simulink model "centralized_FD_basic_01_2017b"  (R2017b)
settings: Solver=VariableStepAuto  StartTime=0.0  StopTime=Tstop  RelTol=1e-3
values from neighbouring files (symbols this model uses):
  faultMag = [0 0 1]    [ProblemData.m]
  faultTime = [1e6 1e6 400]    [ProblemData.m]
  Lambda = diag([0.91 0.91 0.91])    [ProblemData.m]
  noiseRange = [-peakNoise ; +peakNoise]    [ProblemData.m]
  pipeCoeff = [1 1 1]    [ProblemData.m]
  pipeCoeffN = makeParUncertain(pipeCoeff,uncRelative)    [ProblemData.m]
  pipeCross = [5 5 5]*1e-4    [ProblemData.m]
  pipeCrossN = makeParUncertain(pipeCross,uncRelative)    [ProblemData.m]
  pumpACMagRelative = [0.1 0.25]    [ProblemData.m]
  pumpACPeriod = [10 50]    [ProblemData.m]
  pumpDCMag = [1.5 1.5]*1e-3    [ProblemData.m]
  tankCross = [0.156 0.156 0.156]    [ProblemData.m]
  tankCrossN = makeParUncertain(tankCross,uncRelative)    [ProblemData.m]
  tankInit = [0 2.5 5]    [ProblemData.m]
  tankInitN = makeParUncertain(tankInit,uncRelative)    [ProblemData.m]
  tankMax = [10 10 10]    [ProblemData.m]
  tankMaxN = makeParUncertain(tankMax,uncRelative)    [ProblemData.m]
  tankMin = [0 0 0]    [ProblemData.m]
  tankMinN = tankMin    [ProblemData.m]
  Tdelay = 500    [ProblemData.m]
  Ts = 0.01    [ProblemData.m]
(part 1 of 2)
settings Model: Creator=riccardoferrar  LastModifiedBy=TUDelft SID

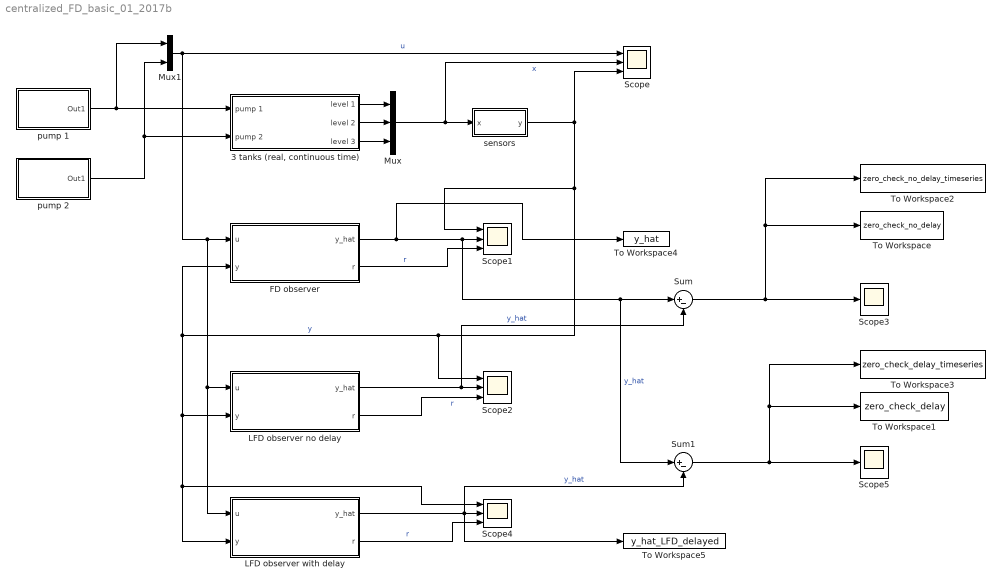
== system centralized_FD_basic_01_2017b ==
  "3 tanks (real, continuous time)" : Subsystem
  FD observer : Subsystem  SystemSampleTime=Ts
  LFD observer no delay : Subsystem  SystemSampleTime=Ts
  LFD observer with delay : Subsystem  SystemSampleTime=Ts
  Mux : Mux  Inputs=3
  Mux1 : Mux  Inputs=2
  Scope{,1..2,4} (4 alike) : Scope  NumInputPorts=3
  Scope3 : Scope
  Scope5 : Scope
  Sum : Sum  Inputs=|+-
  Sum1 : Sum  Inputs=|+-
  To Workspace : ToWorkspace  VariableName=zero_check_no_delay  SampleTime=-1
  To Workspace1 : ToWorkspace  VariableName=zero_check_delay  SampleTime=-1
  To Workspace2 : ToWorkspace  VariableName=zero_check_no_delay_timeseries  SaveFormat=Timeseries  SampleTime=-1
  To Workspace3 : ToWorkspace  VariableName=zero_check_delay_timeseries  SaveFormat=Timeseries  SampleTime=-1
  To Workspace4 : ToWorkspace  VariableName=y_hat  SaveFormat=Timeseries  SampleTime=-1
  To Workspace5 : ToWorkspace  VariableName=y_hat_LFD_delayed  SaveFormat=Timeseries  SampleTime=-1
  pump 1 : Subsystem  mask{pumpIdx=1}
      mask prompts: pumpIdx "Pump number"
  pump 2 : Subsystem  mask{pumpIdx=2}
      mask prompts: pumpIdx "Pump number"
  sensors : Subsystem
  wires:
  pump 1/1(Out1) -> "3 tanks (real, continuous time)"/1(pump 1), Mux1/1
  pump 2/1(Out1) -> Mux1/2, "3 tanks (real, continuous time)"/2(pump 2)
  "3 tanks (real, continuous time)"/1(level 1) -> Mux/1
  "3 tanks (real, continuous time)"/2(level 2) -> Mux/2
  "3 tanks (real, continuous time)"/3(level 3) -> Mux/3
  Mux1/1 -> LFD observer with delay/1(u), LFD observer no delay/1(u), FD observer/1(u), Scope/1  "u"
  sensors/1(y) -> Scope/3, Scope1/1, Scope2/1, Scope4/1, LFD observer with delay/2(y), LFD observer no delay/2(y), FD observer/2(y)  "y"
  FD observer/1(y_hat) -> To Workspace4/1, Sum1/1, Sum/1, Scope1/2  "y_hat"
  FD observer/2(r) -> Scope1/3  "r"
  Mux/1 -> Scope/2, sensors/1(x)  "x"
  LFD observer no delay/1(y_hat) -> Sum/2, Scope2/2  "y_hat"
  LFD observer no delay/2(r) -> Scope2/3  "r"
  Sum/1 -> To Workspace2/1, To Workspace/1, Scope3/1
  LFD observer with delay/1(y_hat) -> To Workspace5/1, Scope4/2, Sum1/2  "y_hat"
  LFD observer with delay/2(r) -> Scope4/3  "r"
  Sum1/1 -> To Workspace3/1, To Workspace1/1, Scope5/1

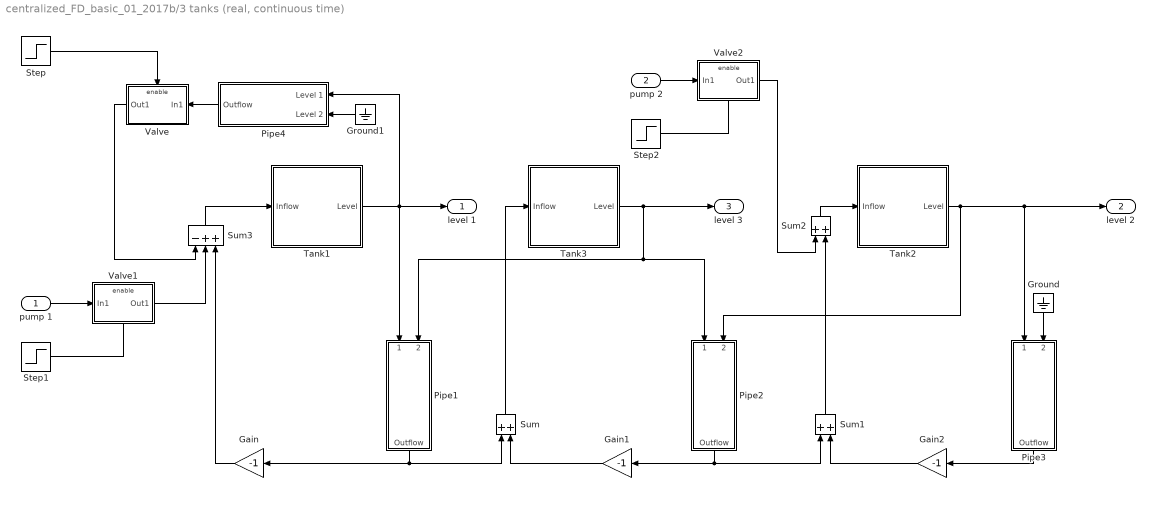
== system centralized_FD_basic_01_2017b/3 tanks (real, continuous time) ==
  pump 1 : Inport
  pump 2 : Inport  Port=2
  Gain : Gain  Gain=-1
  Gain1 : Gain  Gain=-1
  Gain2 : Gain  Gain=-1
  Ground : Ground
  Ground1 : Ground
  Pipe1 : Subsystem  mask(Connection Pipe){S_p=pipeCross(1), c_o=pipeCoeff(1)}
      mask prompts: S_p "Pipe cross-section [m^2]"; c_o "Outflow coefficient"
      mask help:
      | Connection pipe between two tanks.
      | The pipe cross-section and the outflow coefficient are mask block parameters.
      mask Help:
      | Enter the pipe cross-section [S_p] and the outflow coefficient [c_o] in the block dialog parameter fields.
      | 
      | The block generates the pipe's flow-rate. The input signals are the level of fluid into both the tanks, connected by the pipe. If the level in the first tank is bigger than the level in the second one, the fluid flow from the first to the second tank, else in the opposite way.
      mask Display: image(imread('pipe.jpg'));
  Pipe2 : Subsystem  mask(Connection Pipe){S_p=pipeCross(2), c_o=pipeCoeff(2)}
      mask prompts: S_p "Pipe cross-section [m^2]"; c_o "Outflow coefficient"
      mask help:
      | Connection pipe between two tanks.
      | The pipe cross-section and the outflow coefficient are mask block parameters.
      mask Help:
      | Enter the pipe cross-section [S_p] and the outflow coefficient [c_o] in the block dialog parameter fields.
      | 
      | The block generates the pipe's flow-rate. The input signals are the level of fluid into both the tanks, connected by the pipe. If the level in the first tank is bigger than the level in the second one, the fluid flow from the first to the second tank, else in the opposite way.
      mask Display: image(imread('pipe.jpg'));
  Pipe3 : Subsystem  mask(Connection Pipe){S_p=pipeCross(3), c_o=pipeCoeff(3)}
      mask prompts: S_p "Pipe cross-section [m^2]"; c_o "Outflow coefficient"
      mask help:
      | Connection pipe between two tanks.
      | The pipe cross-section and the outflow coefficient are mask block parameters.
      mask Help:
      | Enter the pipe cross-section [S_p] and the outflow coefficient [c_o] in the block dialog parameter fields.
      | 
      | The block generates the pipe's flow-rate. The input signals are the level of fluid into both the tanks, connected by the pipe. If the level in the first tank is bigger than the level in the second one, the fluid flow from the first to the second tank, else in the opposite way.
      mask Display: image(imread('pipe.jpg'));
  Pipe4 : Subsystem  mask(Connection Pipe){S_p=faultMag(2), c_o=1}
      mask prompts: S_p "Pipe cross-section [m^2]"; c_o "Outflow coefficient"
      mask help:
      | Connection pipe between two tanks.
      | The pipe cross-section and the outflow coefficient are mask block parameters.
      mask Help:
      | Enter the pipe cross-section [S_p] and the outflow coefficient [c_o] in the block dialog parameter fields.
      | 
      | The block generates the pipe's flow-rate. The input signals are the level of fluid into both the tanks, connected by the pipe. If the level in the first tank is bigger than the level in the second one, the fluid flow from the first to the second tank, else in the opposite way.
      mask Display: image(imread('pipe.jpg'));
  Step : Step  Time=faultTime(2)  SampleTime=0
  Step1 : Step  Time=faultTime(1)  Before=1  After=1-faultMag(1)  SampleTime=0
  Step2 : Step  Time=faultTime(3)  Before=1  After=1-faultMag(3)  SampleTime=0
  Sum : Sum
  Sum1 : Sum
  Sum2 : Sum
  Sum3 : Sum  Inputs=-++
  Tank1 : Subsystem  mask(Tank system){S=tankCross(1), x_0=tankInit(1), max_level=tankMax(1), min_level=tankMin(1)}
      mask prompts: S "Tank cross-section [m^2]"; x_0 "Initial fluid level [m"; max_level "Maximum fluid level [m]"; min_level "Minimum fluid level [m]"
      mask help:
      | Model of  a simple tank system. The input is a fluid flow-rate (may be positive or negative), the output is the fluid level in the tank.
      |
      | The tank cross-section, the initial, minimum and maximum fluid level are mask block parameters.
      mask Help:
      | Enter the tank cross-section, the initial, minimum, maximum fluid level in the block dialog parameter fields.
      | 
      | The block models a simple tank system. The input is the fluid flow-rate (positive or negative) that feeds the system; the output is the fluid level in the tank.
      mask Display: image(imread('tank.jpg'));
  Tank2 : Subsystem  mask(Tank system){S=tankCross(2), x_0=tankInit(2), max_level=tankMax(2), min_level=tankMin(2)}
      mask prompts: S "Tank cross-section [m^2]"; x_0 "Initial fluid level [m"; max_level "Maximum fluid level [m]"; min_level "Minimum fluid level [m]"
      mask help:
      | Model of  a simple tank system. The input is a fluid flow-rate (may be positive or negative), the output is the fluid level in the tank.
      |
      | The tank cross-section, the initial, minimum and maximum fluid level are mask block parameters.
      mask Help:
      | Enter the tank cross-section, the initial, minimum, maximum fluid level in the block dialog parameter fields.
      | 
      | The block models a simple tank system. The input is the fluid flow-rate (positive or negative) that feeds the system; the output is the fluid level in the tank.
      mask Display: image(imread('tank.jpg'));
  Tank3 : Subsystem  mask(Tank system){S=tankCross(3), x_0=tankInit(3), max_level=tankMax(3), min_level=tankMin(3)}
      mask prompts: S "Tank cross-section [m^2]"; x_0 "Initial fluid level [m"; max_level "Maximum fluid level [m]"; min_level "Minimum fluid level [m]"
      mask help:
      | Model of  a simple tank system. The input is a fluid flow-rate (may be positive or negative), the output is the fluid level in the tank.
      |
      | The tank cross-section, the initial, minimum and maximum fluid level are mask block parameters.
      mask Help:
      | Enter the tank cross-section, the initial, minimum, maximum fluid level in the block dialog parameter fields.
      | 
      | The block models a simple tank system. The input is the fluid flow-rate (positive or negative) that feeds the system; the output is the fluid level in the tank.
      mask Display: image(imread('tank.jpg'));
  Valve : Subsystem  TreatAsAtomicUnit=on  mask(Valve subsystem){}
      mask help: Model of a valve. When the control signal is greather then 0, the output is equal to the input. Otherwise, the output is 0.
      mask Display: image(imread('valve.jpg'))
  Valve1 : Subsystem  TreatAsAtomicUnit=on  mask(Valve subsystem){}
      mask help: Model of a valve. When the control signal is greather then 0, the output is equal to the input. Otherwise, the output is 0.
      mask Display: image(imread('valve.jpg'))
  Valve2 : Subsystem  TreatAsAtomicUnit=on  mask(Valve subsystem){}
      mask help: Model of a valve. When the control signal is greather then 0, the output is equal to the input. Otherwise, the output is 0.
      mask Display: image(imread('valve.jpg'))
  level 1 : Outport
  level 2 : Outport  Port=2
  level 3 : Outport  Port=3
  wires:
  Sum/1 -> Tank3/1(Inflow)
  Gain1/1 -> Sum/2
  Pipe2/1(Outflow) -> Sum1/1, Gain1/1
  Gain/1 -> Sum3/3
  Tank2/1(Level) -> level 2/1, Pipe3/1(Level 1), Pipe2/2(Level 2)
  Sum1/1 -> Sum2/2
  Gain2/1 -> Sum1/2
  Pipe3/1(Outflow) -> Gain2/1
  Tank1/1(Level) -> Pipe1/1(Level 1), Pipe4/1(Level 1), level 1/1
  Tank3/1(Level) -> level 3/1, Pipe2/1(Level 1), Pipe1/2(Level 2)
  Pipe1/1(Outflow) -> Gain/1, Sum/1
  Valve2/1(Out1) -> Sum2/1
  Sum2/1 -> Tank2/1(Inflow)
  Sum3/1 -> Tank1/1(Inflow)
  Ground/1 -> Pipe3/2(Level 2)
  Ground1/1 -> Pipe4/2(Level 2)
  Pipe4/1(Outflow) -> Valve/1(In1)
  Valve/1(Out1) -> Sum3/1
  Step/1 -> Valve/Enable
  pump 1/1 -> Valve1/1(In1)
  Valve1/1(Out1) -> Sum3/2
  Step1/1 -> Valve1/Enable
  Step2/1 -> Valve2/Enable
  pump 2/1 -> Valve2/1(In1)

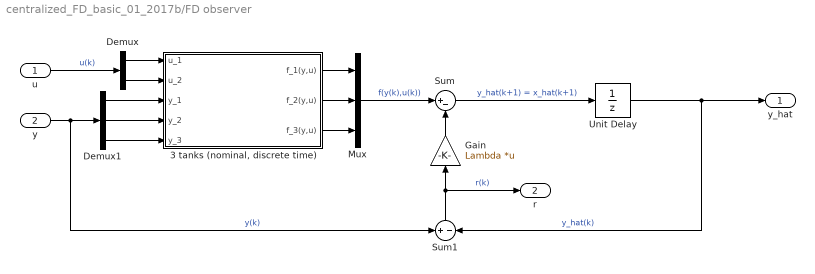
== system centralized_FD_basic_01_2017b/FD observer ==
  u : Inport
  y : Inport  Port=2
  "3 tanks (nominal, discrete time)" : Subsystem
  Demux : Demux  Outputs=2
  Demux1 : Demux  Outputs=3
  Gain : Gain  Gain=Lambda  Multiplication=Matrix(K*u)
  Mux : Mux  Inputs=3
  Sum : Sum  Inputs=|+-
  Sum1 : Sum  Inputs=+|-
  Unit Delay : UnitDelay  InitialCondition=tankInitN  SampleTime=-1
  y_hat : Outport
  r : Outport  Port=2
  wires:
  y/1 -> Sum1/1, Demux1/1  "y(k)"
  Demux1/3 -> "3 tanks (nominal, discrete time)"/5(y_3)
  u/1 -> Demux/1  "u(k)"
  Demux1/2 -> "3 tanks (nominal, discrete time)"/4(y_2)
  Demux/2 -> "3 tanks (nominal, discrete time)"/2(u_2)
  Demux1/1 -> "3 tanks (nominal, discrete time)"/3(y_1)
  Demux/1 -> "3 tanks (nominal, discrete time)"/1(u_1)
  "3 tanks (nominal, discrete time)"/1(f_1(y,u)) -> Mux/1
  "3 tanks (nominal, discrete time)"/2(f_2(y,u)) -> Mux/2
  "3 tanks (nominal, discrete time)"/3(f_3(y,u)) -> Mux/3
  Mux/1 -> Sum/1  "f(y(k),u(k))"
  Sum/1 -> Unit Delay/1  "y_hat(k+1) = x_hat(k+1)"
  Unit Delay/1 -> y_hat/1, Sum1/2  "y_hat(k)"
  Sum1/1 -> r/1, Gain/1  "r(k)"
  Gain/1 -> Sum/2

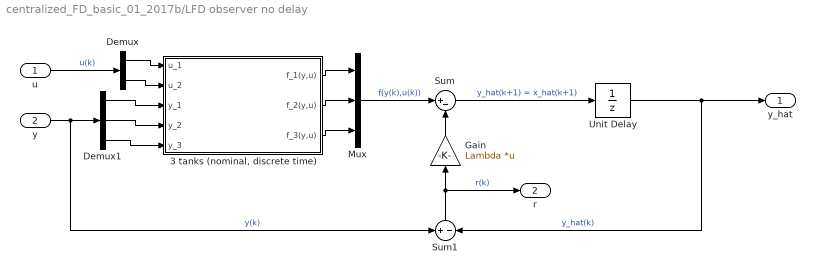
== system centralized_FD_basic_01_2017b/LFD observer no delay ==
  u : Inport
  y : Inport  Port=2
  "3 tanks (nominal, discrete time)" : Subsystem
  Demux : Demux  Outputs=2
  Demux1 : Demux  Outputs=3
  Gain : Gain  Gain=Lambda  Multiplication=Matrix(K*u)
  Mux : Mux  Inputs=3
  Sum : Sum  Inputs=|+-
  Sum1 : Sum  Inputs=+|-
  Unit Delay : UnitDelay  InitialCondition=tankInitN  SampleTime=-1
  y_hat : Outport
  r : Outport  Port=2
  wires:
  y/1 -> Sum1/1, Demux1/1  "y(k)"
  Demux1/3 -> "3 tanks (nominal, discrete time)"/5(y_3)
  u/1 -> Demux/1  "u(k)"
  Demux1/2 -> "3 tanks (nominal, discrete time)"/4(y_2)
  Demux/2 -> "3 tanks (nominal, discrete time)"/2(u_2)
  Demux1/1 -> "3 tanks (nominal, discrete time)"/3(y_1)
  Demux/1 -> "3 tanks (nominal, discrete time)"/1(u_1)
  "3 tanks (nominal, discrete time)"/1(f_1(y,u)) -> Mux/1
  "3 tanks (nominal, discrete time)"/2(f_2(y,u)) -> Mux/2
  "3 tanks (nominal, discrete time)"/3(f_3(y,u)) -> Mux/3
  Mux/1 -> Sum/1  "f(y(k),u(k))"
  Sum/1 -> Unit Delay/1  "y_hat(k+1) = x_hat(k+1)"
  Unit Delay/1 -> y_hat/1, Sum1/2  "y_hat(k)"
  Sum1/1 -> r/1, Gain/1  "r(k)"
  Gain/1 -> Sum/2

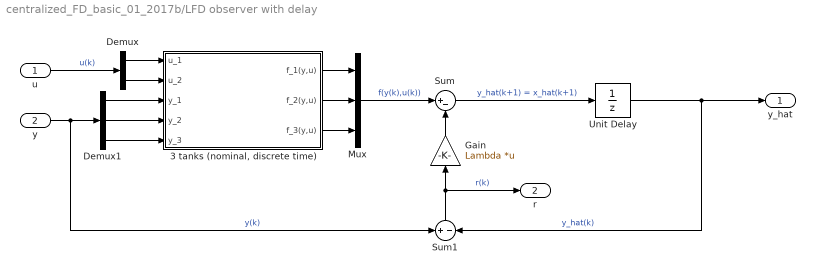
== system centralized_FD_basic_01_2017b/LFD observer with delay ==
  u : Inport
  y : Inport  Port=2
  "3 tanks (nominal, discrete time)" : Subsystem
  Demux : Demux  Outputs=2
  Demux1 : Demux  Outputs=3
  Gain : Gain  Gain=Lambda  Multiplication=Matrix(K*u)
  Mux : Mux  Inputs=3
  Sum : Sum  Inputs=|+-
  Sum1 : Sum  Inputs=+|-
  Unit Delay : UnitDelay  InitialCondition=tankInitN  SampleTime=-1
  y_hat : Outport
  r : Outport  Port=2
  wires:
  y/1 -> Sum1/1, Demux1/1  "y(k)"
  Demux1/3 -> "3 tanks (nominal, discrete time)"/5(y_3)
  u/1 -> Demux/1  "u(k)"
  Demux1/2 -> "3 tanks (nominal, discrete time)"/4(y_2)
  Demux/2 -> "3 tanks (nominal, discrete time)"/2(u_2)
  Demux1/1 -> "3 tanks (nominal, discrete time)"/3(y_1)
  Demux/1 -> "3 tanks (nominal, discrete time)"/1(u_1)
  "3 tanks (nominal, discrete time)"/1(f_1(y,u)) -> Mux/1
  "3 tanks (nominal, discrete time)"/2(f_2(y,u)) -> Mux/2
  "3 tanks (nominal, discrete time)"/3(f_3(y,u)) -> Mux/3
  Mux/1 -> Sum/1  "f(y(k),u(k))"
  Sum/1 -> Unit Delay/1  "y_hat(k+1) = x_hat(k+1)"
  Unit Delay/1 -> y_hat/1, Sum1/2  "y_hat(k)"
  Sum1/1 -> r/1, Gain/1  "r(k)"
  Gain/1 -> Sum/2

== system centralized_FD_basic_01_2017b/pump 1 ==
  Bias : Bias  Bias=1
  Product : Product
  Signal Generator : SignalGenerator  Amplitude=pumpACMagRelative(pumpIdx)  Frequency=1/pumpACPeriod(pumpIdx)  Units=rad/sec
  pump 1 : Constant  Value=pumpDCMag(pumpIdx)
  Out1 : Outport
  wires:
  Product/1 -> Out1/1
  Bias/1 -> Product/1
  pump 1/1 -> Product/2
  Signal Generator/1 -> Bias/1

== system centralized_FD_basic_01_2017b/pump 2 ==
  Bias : Bias  Bias=1
  Product : Product
  Signal Generator : SignalGenerator  Amplitude=pumpACMagRelative(pumpIdx)  Frequency=1/pumpACPeriod(pumpIdx)  Units=rad/sec
  pump 1 : Constant  Value=pumpDCMag(pumpIdx)
  Out1 : Outport
  wires:
  Product/1 -> Out1/1
  Bias/1 -> Product/1
  pump 1/1 -> Product/2
  Signal Generator/1 -> Bias/1

== system centralized_FD_basic_01_2017b/sensors ==
  x : Inport
  Sum : Sum  Inputs=|++
  Uniform Random Number : UniformRandomNumber  Minimum=noiseRange(1,:)  Maximum=noiseRange(2,:)  SampleTime=Ts
  y : Outport
  wires:
  Sum/1 -> y/1
  Uniform Random Number/1 -> Sum/2
  x/1 -> Sum/1

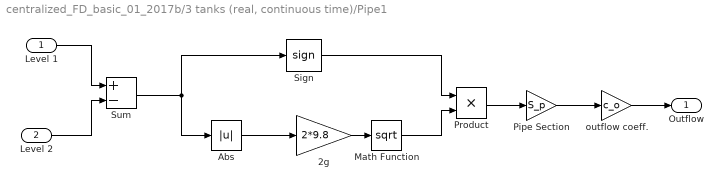
== system centralized_FD_basic_01_2017b/3 tanks (real, continuous time)/Pipe1 ==
  Level 1 : Inport
  Level 2 : Inport  Port=2
  2g : Gain  Gain=2*9.8  SaturateOnIntegerOverflow=on  OutDataTypeStr=Inherit: Same as input  ParamDataTypeStr=Inherit: Same as input
  Abs : Abs  SaturateOnIntegerOverflow=on
  Math Function : Math  Operator=sqrt  SaturateOnIntegerOverflow=on
  Pipe Section : Gain  Gain=S_p  SaturateOnIntegerOverflow=on  OutDataTypeStr=Inherit: Same as input  ParamDataTypeStr=Inherit: Same as input
  Product : Product  SaturateOnIntegerOverflow=on  InputSameDT=on  OutDataTypeStr=Inherit: Same as first input
  Sign : Signum
  Sum : Sum  Inputs=+-  SaturateOnIntegerOverflow=on  InputSameDT=on  OutDataTypeStr=Inherit: Same as first input
  outflow coeff. : Gain  Gain=c_o  SaturateOnIntegerOverflow=on  OutDataTypeStr=Inherit: Same as input  ParamDataTypeStr=Inherit: Same as input
  Outflow : Outport
  wires:
  outflow coeff./1 -> Outflow/1
  Pipe Section/1 -> outflow coeff./1
  Product/1 -> Pipe Section/1
  Sign/1 -> Product/1
  Math Function/1 -> Product/2
  2g/1 -> Math Function/1
  Abs/1 -> 2g/1
  Sum/1 -> Abs/1, Sign/1
  Level 2/1 -> Sum/2
  Level 1/1 -> Sum/1

== system centralized_FD_basic_01_2017b/3 tanks (real, continuous time)/Pipe2 ==
  Level 1 : Inport
  Level 2 : Inport  Port=2
  2g : Gain  Gain=2*9.8  SaturateOnIntegerOverflow=on  OutDataTypeStr=Inherit: Same as input  ParamDataTypeStr=Inherit: Same as input
  Abs : Abs  SaturateOnIntegerOverflow=on
  Math Function : Math  Operator=sqrt  SaturateOnIntegerOverflow=on
  Pipe Section : Gain  Gain=S_p  SaturateOnIntegerOverflow=on  OutDataTypeStr=Inherit: Same as input  ParamDataTypeStr=Inherit: Same as input
  Product : Product  SaturateOnIntegerOverflow=on  InputSameDT=on  OutDataTypeStr=Inherit: Same as first input
  Sign : Signum
  Sum : Sum  Inputs=+-  SaturateOnIntegerOverflow=on  InputSameDT=on  OutDataTypeStr=Inherit: Same as first input
  outflow coeff. : Gain  Gain=c_o  SaturateOnIntegerOverflow=on  OutDataTypeStr=Inherit: Same as input  ParamDataTypeStr=Inherit: Same as input
  Outflow : Outport
  wires:
  outflow coeff./1 -> Outflow/1
  Pipe Section/1 -> outflow coeff./1
  Product/1 -> Pipe Section/1
  Sign/1 -> Product/1
  Math Function/1 -> Product/2
  2g/1 -> Math Function/1
  Abs/1 -> 2g/1
  Sum/1 -> Abs/1, Sign/1
  Level 2/1 -> Sum/2
  Level 1/1 -> Sum/1

== system centralized_FD_basic_01_2017b/3 tanks (real, continuous time)/Pipe3 ==
  Level 1 : Inport
  Level 2 : Inport  Port=2
  2g : Gain  Gain=2*9.8  SaturateOnIntegerOverflow=on  OutDataTypeStr=Inherit: Same as input  ParamDataTypeStr=Inherit: Same as input
  Abs : Abs  SaturateOnIntegerOverflow=on
  Math Function : Math  Operator=sqrt  SaturateOnIntegerOverflow=on
  Pipe Section : Gain  Gain=S_p  SaturateOnIntegerOverflow=on  OutDataTypeStr=Inherit: Same as input  ParamDataTypeStr=Inherit: Same as input
  Product : Product  SaturateOnIntegerOverflow=on  InputSameDT=on  OutDataTypeStr=Inherit: Same as first input
  Sign : Signum
  Sum : Sum  Inputs=+-  SaturateOnIntegerOverflow=on  InputSameDT=on  OutDataTypeStr=Inherit: Same as first input
  outflow coeff. : Gain  Gain=c_o  SaturateOnIntegerOverflow=on  OutDataTypeStr=Inherit: Same as input  ParamDataTypeStr=Inherit: Same as input
  Outflow : Outport
  wires:
  outflow coeff./1 -> Outflow/1
  Pipe Section/1 -> outflow coeff./1
  Product/1 -> Pipe Section/1
  Sign/1 -> Product/1
  Math Function/1 -> Product/2
  2g/1 -> Math Function/1
  Abs/1 -> 2g/1
  Sum/1 -> Abs/1, Sign/1
  Level 2/1 -> Sum/2
  Level 1/1 -> Sum/1

== system centralized_FD_basic_01_2017b/3 tanks (real, continuous time)/Pipe4 ==
  Level 1 : Inport
  Level 2 : Inport  Port=2
  2g : Gain  Gain=2*9.8  SaturateOnIntegerOverflow=on  OutDataTypeStr=Inherit: Same as input  ParamDataTypeStr=Inherit: Same as input
  Abs : Abs  SaturateOnIntegerOverflow=on
  Math Function : Math  Operator=sqrt  SaturateOnIntegerOverflow=on
  Pipe Section : Gain  Gain=S_p  SaturateOnIntegerOverflow=on  OutDataTypeStr=Inherit: Same as input  ParamDataTypeStr=Inherit: Same as input
  Product : Product  SaturateOnIntegerOverflow=on  InputSameDT=on  OutDataTypeStr=Inherit: Same as first input
  Sign : Signum
  Sum : Sum  Inputs=+-  SaturateOnIntegerOverflow=on  InputSameDT=on  OutDataTypeStr=Inherit: Same as first input
  outflow coeff. : Gain  Gain=c_o  SaturateOnIntegerOverflow=on  OutDataTypeStr=Inherit: Same as input  ParamDataTypeStr=Inherit: Same as input
  Outflow : Outport
  wires:
  outflow coeff./1 -> Outflow/1
  Pipe Section/1 -> outflow coeff./1
  Product/1 -> Pipe Section/1
  Sign/1 -> Product/1
  Math Function/1 -> Product/2
  2g/1 -> Math Function/1
  Abs/1 -> 2g/1
  Sum/1 -> Abs/1, Sign/1
  Level 2/1 -> Sum/2
  Level 1/1 -> Sum/1

== system centralized_FD_basic_01_2017b/3 tanks (real, continuous time)/Tank1 ==
  Inflow : Inport
  Initial Level : Constant  Value=x_0
  Integrator : Integrator  InitialConditionSource=external  LimitOutput=on  UpperSaturationLimit=max_level  LowerSaturationLimit=min_level
  Tank Section : Gain  Gain=1/S  SaturateOnIntegerOverflow=on  OutDataTypeStr=Inherit: Same as input  ParamDataTypeStr=Inherit: Same as input
  Level : Outport  InitialOutput=0
  wires:
  Integrator/1 -> Level/1
  Initial Level/1 -> Integrator/2
  Tank Section/1 -> Integrator/1
  Inflow/1 -> Tank Section/1

== system centralized_FD_basic_01_2017b/3 tanks (real, continuous time)/Tank2 ==
  Inflow : Inport
  Initial Level : Constant  Value=x_0
  Integrator : Integrator  InitialConditionSource=external  LimitOutput=on  UpperSaturationLimit=max_level  LowerSaturationLimit=min_level
  Tank Section : Gain  Gain=1/S  SaturateOnIntegerOverflow=on  OutDataTypeStr=Inherit: Same as input  ParamDataTypeStr=Inherit: Same as input
  Level : Outport  InitialOutput=0
  wires:
  Integrator/1 -> Level/1
  Initial Level/1 -> Integrator/2
  Tank Section/1 -> Integrator/1
  Inflow/1 -> Tank Section/1

== system centralized_FD_basic_01_2017b/3 tanks (real, continuous time)/Tank3 ==
  Inflow : Inport
  Initial Level : Constant  Value=x_0
  Integrator : Integrator  InitialConditionSource=external  LimitOutput=on  UpperSaturationLimit=max_level  LowerSaturationLimit=min_level
  Tank Section : Gain  Gain=1/S  SaturateOnIntegerOverflow=on  OutDataTypeStr=Inherit: Same as input  ParamDataTypeStr=Inherit: Same as input
  Level : Outport  InitialOutput=0
  wires:
  Integrator/1 -> Level/1
  Initial Level/1 -> Integrator/2
  Tank Section/1 -> Integrator/1
  Inflow/1 -> Tank Section/1

== system centralized_FD_basic_01_2017b/3 tanks (real, continuous time)/Valve ==
  In1 : Inport
  Enable : EnablePort  StatesWhenEnabling=reset  ShowOutputPort=on
  Product : Product  SaturateOnIntegerOverflow=on  InputSameDT=on  OutDataTypeStr=Inherit: Same as first input
  Saturation : Saturate  UpperLimit=1.0  LowerLimit=0.0
  Out1 : Outport  OutputWhenDisabled=reset  InitialOutput=0
  wires:
  Enable/1 -> Saturation/1
  Saturation/1 -> Product/1
  In1/1 -> Product/2
  Product/1 -> Out1/1

== system centralized_FD_basic_01_2017b/3 tanks (real, continuous time)/Valve1 ==
  In1 : Inport
  Enable : EnablePort  StatesWhenEnabling=reset  ShowOutputPort=on
  Product : Product  SaturateOnIntegerOverflow=on  InputSameDT=on  OutDataTypeStr=Inherit: Same as first input
  Saturation : Saturate  UpperLimit=1.0  LowerLimit=0.0
  Out1 : Outport  OutputWhenDisabled=reset  InitialOutput=0
  wires:
  Enable/1 -> Saturation/1
  Saturation/1 -> Product/1
  In1/1 -> Product/2
  Product/1 -> Out1/1

== system centralized_FD_basic_01_2017b/3 tanks (real, continuous time)/Valve2 ==
  In1 : Inport
  Enable : EnablePort  StatesWhenEnabling=reset  ShowOutputPort=on
  Product : Product  SaturateOnIntegerOverflow=on  InputSameDT=on  OutDataTypeStr=Inherit: Same as first input
  Saturation : Saturate  UpperLimit=1.0  LowerLimit=0.0
  Out1 : Outport  OutputWhenDisabled=reset  InitialOutput=0
  wires:
  Enable/1 -> Saturation/1
  Saturation/1 -> Product/1
  In1/1 -> Product/2
  Product/1 -> Out1/1

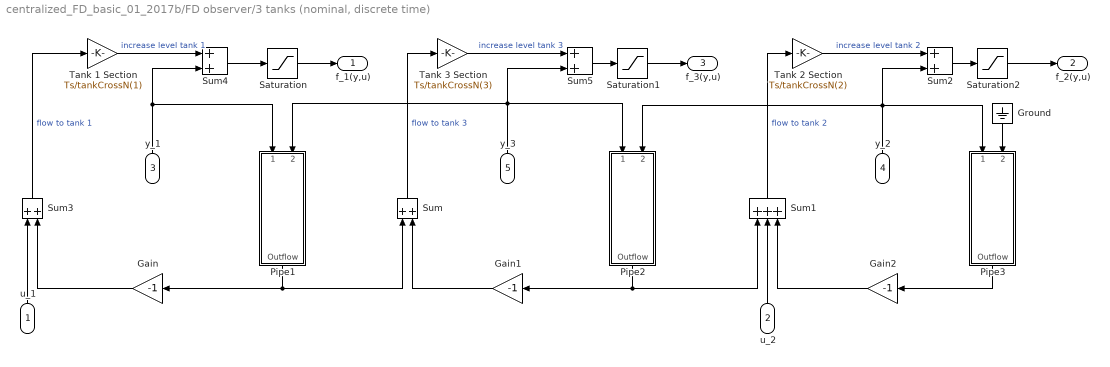
== system centralized_FD_basic_01_2017b/FD observer/3 tanks (nominal, discrete time) ==
  u_1 : Inport
  u_2 : Inport  Port=2
  y_1 : Inport  Port=3
  y_2 : Inport  Port=4
  y_3 : Inport  Port=5
  Gain : Gain  Gain=-1
  Gain1 : Gain  Gain=-1
  Gain2 : Gain  Gain=-1
  Ground : Ground
  Pipe1 : Subsystem  mask(Connection Pipe){S_p=pipeCrossN(1), c_o=pipeCoeffN(1)}
      mask prompts: S_p "Pipe cross-section [m^2]"; c_o "Outflow coefficient"
      mask help:
      | Connection pipe between two tanks.
      | The pipe cross-section and the outflow coefficient are mask block parameters.
      mask Help:
      | Enter the pipe cross-section [S_p] and the outflow coefficient [c_o] in the block dialog parameter fields.
      | 
      | The block generates the pipe's flow-rate. The input signals are the level of fluid into both the tanks, connected by the pipe. If the level in the first tank is bigger than the level in the second one, the fluid flow from the first to the second tank, else in the opposite way.
      mask Display: image(imread('pipe.jpg'));
  Pipe2 : Subsystem  mask(Connection Pipe){S_p=pipeCrossN(2), c_o=pipeCoeffN(2)}
      mask prompts: S_p "Pipe cross-section [m^2]"; c_o "Outflow coefficient"
      mask help:
      | Connection pipe between two tanks.
      | The pipe cross-section and the outflow coefficient are mask block parameters.
      mask Help:
      | Enter the pipe cross-section [S_p] and the outflow coefficient [c_o] in the block dialog parameter fields.
      | 
      | The block generates the pipe's flow-rate. The input signals are the level of fluid into both the tanks, connected by the pipe. If the level in the first tank is bigger than the level in the second one, the fluid flow from the first to the second tank, else in the opposite way.
      mask Display: image(imread('pipe.jpg'));
  Pipe3 : Subsystem  mask(Connection Pipe){S_p=pipeCrossN(3), c_o=pipeCoeffN(3)}
      mask prompts: S_p "Pipe cross-section [m^2]"; c_o "Outflow coefficient"
      mask help:
      | Connection pipe between two tanks.
      | The pipe cross-section and the outflow coefficient are mask block parameters.
      mask Help:
      | Enter the pipe cross-section [S_p] and the outflow coefficient [c_o] in the block dialog parameter fields.
      | 
      | The block generates the pipe's flow-rate. The input signals are the level of fluid into both the tanks, connected by the pipe. If the level in the first tank is bigger than the level in the second one, the fluid flow from the first to the second tank, else in the opposite way.
      mask Display: image(imread('pipe.jpg'));
  Saturation : Saturate  UpperLimit=tankMaxN(1)  LowerLimit=tankMinN(1)
  Saturation1 : Saturate  UpperLimit=tankMaxN(3)  LowerLimit=tankMinN(3)
  Saturation2 : Saturate  UpperLimit=tankMaxN(2)  LowerLimit=tankMinN(2)
  Sum{,2..5} (5 alike) : Sum
  Sum1 : Sum  Inputs=+++
  Tank 1 Section : Gain  Gain=Ts/tankCrossN(1)  SaturateOnIntegerOverflow=on  OutDataTypeStr=Inherit: Same as input  ParamDataTypeStr=Inherit: Same as input
  Tank 2 Section : Gain  Gain=Ts/tankCrossN(2)  SaturateOnIntegerOverflow=on  OutDataTypeStr=Inherit: Same as input  ParamDataTypeStr=Inherit: Same as input
  Tank 3 Section : Gain  Gain=Ts/tankCrossN(3)  SaturateOnIntegerOverflow=on  OutDataTypeStr=Inherit: Same as input  ParamDataTypeStr=Inherit: Same as input
  f_1(y,u) : Outport
  f_2(y,u) : Outport  Port=2
  f_3(y,u) : Outport  Port=3
  wires:
  Sum/1 -> Tank 3 Section/1  "flow to tank 3"
  Gain1/1 -> Sum/2
  Pipe2/1(Outflow) -> Sum1/1, Gain1/1
  Gain/1 -> Sum3/2
  Sum1/1 -> Tank 2 Section/1  "flow to tank 2"
  Gain2/1 -> Sum1/3
  Pipe3/1(Outflow) -> Gain2/1
  y_1/1 -> Pipe1/1(Level 1), Sum4/2
  y_3/1 -> Pipe2/1(Level 1), Sum5/2, Pipe1/2(Level 2)
  Pipe1/1(Outflow) -> Sum/1, Gain/1
  Sum3/1 -> Tank 1 Section/1  "flow to tank 1"
  Ground/1 -> Pipe3/2(Level 2)
  u_1/1 -> Sum3/1
  Tank 1 Section/1 -> Sum4/1  "increase level tank 1"
  Sum4/1 -> Saturation/1
  Saturation/1 -> f_1(y,u)/1
  Sum5/1 -> Saturation1/1
  Saturation1/1 -> f_3(y,u)/1
  Tank 3 Section/1 -> Sum5/1  "increase level tank 3"
  u_2/1 -> Sum1/2
  Saturation2/1 -> f_2(y,u)/1
  Sum2/1 -> Saturation2/1
  y_2/1 -> Pipe2/2(Level 2), Sum2/2, Pipe3/1(Level 1)
  Tank 2 Section/1 -> Sum2/1  "increase level tank 2"

== system centralized_FD_basic_01_2017b/LFD observer no delay/3 tanks (nominal, discrete time) ==
  u_1 : Inport
  u_2 : Inport  Port=2
  y_1 : Inport  Port=3
  y_2 : Inport  Port=4
  y_3 : Inport  Port=5
  Subsystem : Subsystem
  Subsystem1 : Subsystem
  f_1(y,u) : Outport
  f_2(y,u) : Outport  Port=2
  f_3(y,u) : Outport  Port=3
  wires:
  u_1/1 -> Subsystem/1(u_1)
  y_1/1 -> Subsystem/2(y_1)
  y_3/1 -> Subsystem1/3(y_3), Subsystem/3(y_3)
  y_2/1 -> Subsystem1/2(y_2), Subsystem/4(y_2)
  u_2/1 -> Subsystem1/1(u_2)
  Subsystem/1(f_1(y,u)) -> f_1(y,u)/1
  Subsystem/2(f_3(y,u)) -> f_3(y,u)/1
  Subsystem1/1(f_2(y,u)) -> f_2(y,u)/1

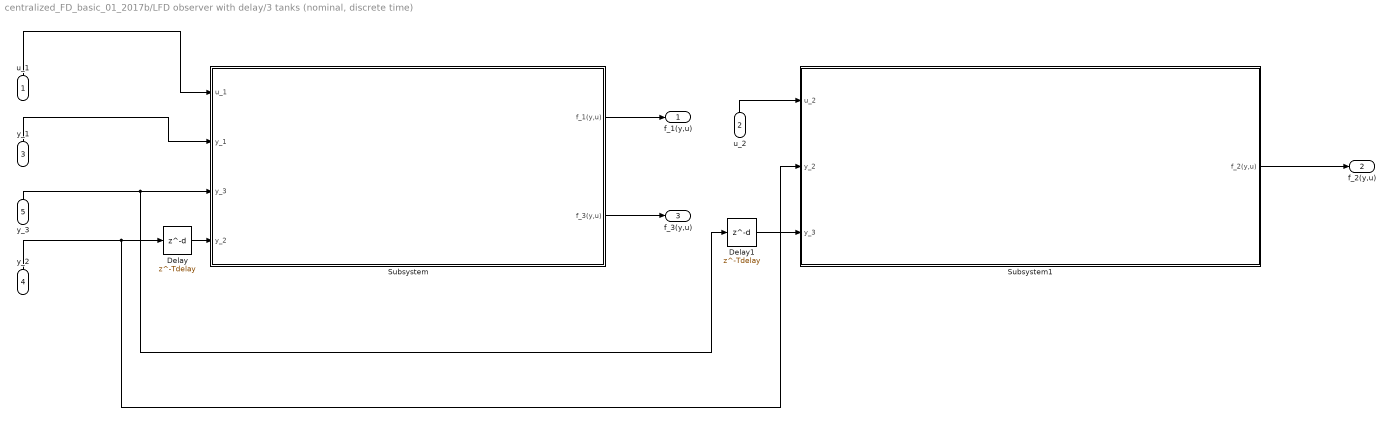
== system centralized_FD_basic_01_2017b/LFD observer with delay/3 tanks (nominal, discrete time) ==
  u_1 : Inport
  u_2 : Inport  Port=2
  y_1 : Inport  Port=3
  y_2 : Inport  Port=4
  y_3 : Inport  Port=5
  Delay : Delay  DelayLength=Tdelay  InitialCondition=0
  Delay1 : Delay  DelayLength=Tdelay  InitialCondition=0
  Subsystem : Subsystem
  Subsystem1 : Subsystem
  f_1(y,u) : Outport
  f_2(y,u) : Outport  Port=2
  f_3(y,u) : Outport  Port=3
  wires:
  u_1/1 -> Subsystem/1(u_1)
  y_1/1 -> Subsystem/2(y_1)
  u_2/1 -> Subsystem1/1(u_2)
  y_2/1 -> Delay/1, Subsystem1/2(y_2)
  y_3/1 -> Delay1/1, Subsystem/3(y_3)
  Subsystem/1(f_1(y,u)) -> f_1(y,u)/1
  Subsystem/2(f_3(y,u)) -> f_3(y,u)/1
  Subsystem1/1(f_2(y,u)) -> f_2(y,u)/1
  Delay1/1 -> Subsystem1/3(y_3)
  Delay/1 -> Subsystem/4(y_2)

== system centralized_FD_basic_01_2017b/FD observer/3 tanks (nominal, discrete time)/Pipe1 ==
  Level 1 : Inport
  Level 2 : Inport  Port=2
  2g : Gain  Gain=2*9.8  SaturateOnIntegerOverflow=on  OutDataTypeStr=Inherit: Same as input  ParamDataTypeStr=Inherit: Same as input
  Abs : Abs  SaturateOnIntegerOverflow=on
  Math Function : Math  Operator=sqrt  SaturateOnIntegerOverflow=on
  Pipe Section : Gain  Gain=S_p  SaturateOnIntegerOverflow=on  OutDataTypeStr=Inherit: Same as input  ParamDataTypeStr=Inherit: Same as input
  Product : Product  SaturateOnIntegerOverflow=on  InputSameDT=on  OutDataTypeStr=Inherit: Same as first input
  Sign : Signum
  Sum : Sum  Inputs=+-  SaturateOnIntegerOverflow=on  InputSameDT=on  OutDataTypeStr=Inherit: Same as first input
  outflow coeff. : Gain  Gain=c_o  SaturateOnIntegerOverflow=on  OutDataTypeStr=Inherit: Same as input  ParamDataTypeStr=Inherit: Same as input
  Outflow : Outport
  wires:
  outflow coeff./1 -> Outflow/1
  Pipe Section/1 -> outflow coeff./1
  Product/1 -> Pipe Section/1
  Sign/1 -> Product/1
  Math Function/1 -> Product/2
  2g/1 -> Math Function/1
  Abs/1 -> 2g/1
  Sum/1 -> Abs/1, Sign/1
  Level 2/1 -> Sum/2
  Level 1/1 -> Sum/1

== system centralized_FD_basic_01_2017b/FD observer/3 tanks (nominal, discrete time)/Pipe2 ==
  Level 1 : Inport
  Level 2 : Inport  Port=2
  2g : Gain  Gain=2*9.8  SaturateOnIntegerOverflow=on  OutDataTypeStr=Inherit: Same as input  ParamDataTypeStr=Inherit: Same as input
  Abs : Abs  SaturateOnIntegerOverflow=on
  Math Function : Math  Operator=sqrt  SaturateOnIntegerOverflow=on
  Pipe Section : Gain  Gain=S_p  SaturateOnIntegerOverflow=on  OutDataTypeStr=Inherit: Same as input  ParamDataTypeStr=Inherit: Same as input
  Product : Product  SaturateOnIntegerOverflow=on  InputSameDT=on  OutDataTypeStr=Inherit: Same as first input
  Sign : Signum
  Sum : Sum  Inputs=+-  SaturateOnIntegerOverflow=on  InputSameDT=on  OutDataTypeStr=Inherit: Same as first input
  outflow coeff. : Gain  Gain=c_o  SaturateOnIntegerOverflow=on  OutDataTypeStr=Inherit: Same as input  ParamDataTypeStr=Inherit: Same as input
  Outflow : Outport
  wires:
  outflow coeff./1 -> Outflow/1
  Pipe Section/1 -> outflow coeff./1
  Product/1 -> Pipe Section/1
  Sign/1 -> Product/1
  Math Function/1 -> Product/2
  2g/1 -> Math Function/1
  Abs/1 -> 2g/1
  Sum/1 -> Abs/1, Sign/1
  Level 2/1 -> Sum/2
  Level 1/1 -> Sum/1

== system centralized_FD_basic_01_2017b/FD observer/3 tanks (nominal, discrete time)/Pipe3 ==
  Level 1 : Inport
  Level 2 : Inport  Port=2
  2g : Gain  Gain=2*9.8  SaturateOnIntegerOverflow=on  OutDataTypeStr=Inherit: Same as input  ParamDataTypeStr=Inherit: Same as input
  Abs : Abs  SaturateOnIntegerOverflow=on
  Math Function : Math  Operator=sqrt  SaturateOnIntegerOverflow=on
  Pipe Section : Gain  Gain=S_p  SaturateOnIntegerOverflow=on  OutDataTypeStr=Inherit: Same as input  ParamDataTypeStr=Inherit: Same as input
  Product : Product  SaturateOnIntegerOverflow=on  InputSameDT=on  OutDataTypeStr=Inherit: Same as first input
  Sign : Signum
  Sum : Sum  Inputs=+-  SaturateOnIntegerOverflow=on  InputSameDT=on  OutDataTypeStr=Inherit: Same as first input
  outflow coeff. : Gain  Gain=c_o  SaturateOnIntegerOverflow=on  OutDataTypeStr=Inherit: Same as input  ParamDataTypeStr=Inherit: Same as input
  Outflow : Outport
  wires:
  outflow coeff./1 -> Outflow/1
  Pipe Section/1 -> outflow coeff./1
  Product/1 -> Pipe Section/1
  Sign/1 -> Product/1
  Math Function/1 -> Product/2
  2g/1 -> Math Function/1
  Abs/1 -> 2g/1
  Sum/1 -> Abs/1, Sign/1
  Level 2/1 -> Sum/2
  Level 1/1 -> Sum/1

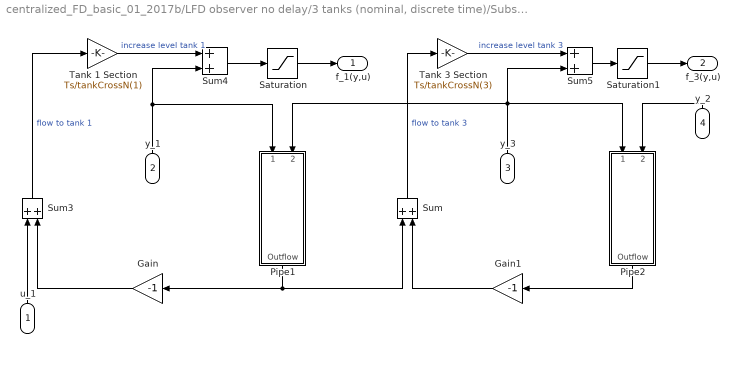
== system centralized_FD_basic_01_2017b/LFD observer no delay/3 tanks (nominal, discrete time)/Subsystem ==
  u_1 : Inport
  y_1 : Inport  Port=2
  y_3 : Inport  Port=3
  y_2 : Inport  Port=4
  Gain : Gain  Gain=-1
  Gain1 : Gain  Gain=-1
  Pipe1 : Subsystem  mask(Connection Pipe){S_p=pipeCrossN(1), c_o=pipeCoeffN(1)}
      mask prompts: S_p "Pipe cross-section [m^2]"; c_o "Outflow coefficient"
      mask help:
      | Connection pipe between two tanks.
      | The pipe cross-section and the outflow coefficient are mask block parameters.
      mask Help:
      | Enter the pipe cross-section [S_p] and the outflow coefficient [c_o] in the block dialog parameter fields.
      | 
      | The block generates the pipe's flow-rate. The input signals are the level of fluid into both the tanks, connected by the pipe. If the level in the first tank is bigger than the level in the second one, the fluid flow from the first to the second tank, else in the opposite way.
      mask Display: image(imread('pipe.jpg'));
  Pipe2 : Subsystem  mask(Connection Pipe){S_p=pipeCrossN(2), c_o=pipeCoeffN(2)}
      mask prompts: S_p "Pipe cross-section [m^2]"; c_o "Outflow coefficient"
      mask help:
      | Connection pipe between two tanks.
      | The pipe cross-section and the outflow coefficient are mask block parameters.
      mask Help:
      | Enter the pipe cross-section [S_p] and the outflow coefficient [c_o] in the block dialog parameter fields.
      | 
      | The block generates the pipe's flow-rate. The input signals are the level of fluid into both the tanks, connected by the pipe. If the level in the first tank is bigger than the level in the second one, the fluid flow from the first to the second tank, else in the opposite way.
      mask Display: image(imread('pipe.jpg'));
  Saturation : Saturate  UpperLimit=tankMaxN(1)  LowerLimit=tankMinN(1)
  Saturation1 : Saturate  UpperLimit=tankMaxN(3)  LowerLimit=tankMinN(3)
  Sum{,3..5} (4 alike) : Sum
  Tank 1 Section : Gain  Gain=Ts/tankCrossN(1)  SaturateOnIntegerOverflow=on  OutDataTypeStr=Inherit: Same as input  ParamDataTypeStr=Inherit: Same as input
  Tank 3 Section : Gain  Gain=Ts/tankCrossN(3)  SaturateOnIntegerOverflow=on  OutDataTypeStr=Inherit: Same as input  ParamDataTypeStr=Inherit: Same as input
  f_1(y,u) : Outport
  f_3(y,u) : Outport  Port=2
  wires:
  Saturation1/1 -> f_3(y,u)/1
  Sum3/1 -> Tank 1 Section/1  "flow to tank 1"
  y_2/1 -> Pipe2/2(Level 2)
  Pipe2/1(Outflow) -> Gain1/1
  Tank 3 Section/1 -> Sum5/1  "increase level tank 3"
  Pipe1/1(Outflow) -> Sum/1, Gain/1
  Tank 1 Section/1 -> Sum4/1  "increase level tank 1"
  u_1/1 -> Sum3/1
  Saturation/1 -> f_1(y,u)/1
  Gain/1 -> Sum3/2
  Sum4/1 -> Saturation/1
  y_1/1 -> Pipe1/1(Level 1), Sum4/2
  Sum5/1 -> Saturation1/1
  Sum/1 -> Tank 3 Section/1  "flow to tank 3"
  Gain1/1 -> Sum/2
  y_3/1 -> Pipe2/1(Level 1), Sum5/2, Pipe1/2(Level 2)

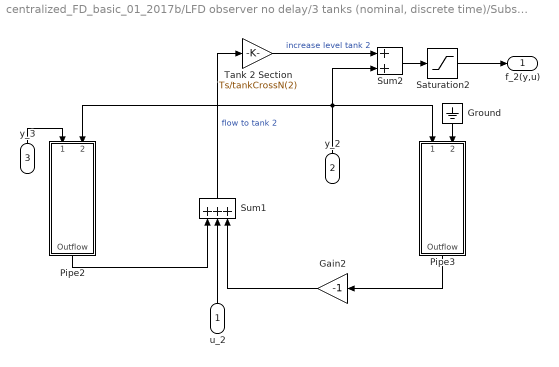
== system centralized_FD_basic_01_2017b/LFD observer no delay/3 tanks (nominal, discrete time)/Subsystem1 ==
  u_2 : Inport
  y_2 : Inport  Port=2
  y_3 : Inport  Port=3
  Gain2 : Gain  Gain=-1
  Ground : Ground
  Pipe2 : Subsystem  mask(Connection Pipe){S_p=pipeCrossN(2), c_o=pipeCoeffN(2)}
      mask prompts: S_p "Pipe cross-section [m^2]"; c_o "Outflow coefficient"
      mask help:
      | Connection pipe between two tanks.
      | The pipe cross-section and the outflow coefficient are mask block parameters.
      mask Help:
      | Enter the pipe cross-section [S_p] and the outflow coefficient [c_o] in the block dialog parameter fields.
      | 
      | The block generates the pipe's flow-rate. The input signals are the level of fluid into both the tanks, connected by the pipe. If the level in the first tank is bigger than the level in the second one, the fluid flow from the first to the second tank, else in the opposite way.
      mask Display: image(imread('pipe.jpg'));
  Pipe3 : Subsystem  mask(Connection Pipe){S_p=pipeCrossN(3), c_o=pipeCoeffN(3)}
      mask prompts: S_p "Pipe cross-section [m^2]"; c_o "Outflow coefficient"
      mask help:
      | Connection pipe between two tanks.
      | The pipe cross-section and the outflow coefficient are mask block parameters.
      mask Help:
      | Enter the pipe cross-section [S_p] and the outflow coefficient [c_o] in the block dialog parameter fields.
      | 
      | The block generates the pipe's flow-rate. The input signals are the level of fluid into both the tanks, connected by the pipe. If the level in the first tank is bigger than the level in the second one, the fluid flow from the first to the second tank, else in the opposite way.
      mask Display: image(imread('pipe.jpg'));
  Saturation2 : Saturate  UpperLimit=tankMaxN(2)  LowerLimit=tankMinN(2)
  Sum1 : Sum  Inputs=+++
  Sum2 : Sum
  Tank 2 Section : Gain  Gain=Ts/tankCrossN(2)  SaturateOnIntegerOverflow=on  OutDataTypeStr=Inherit: Same as input  ParamDataTypeStr=Inherit: Same as input
  f_2(y,u) : Outport
  wires:
  Tank 2 Section/1 -> Sum2/1  "increase level tank 2"
  y_2/1 -> Pipe2/2(Level 2), Sum2/2, Pipe3/1(Level 1)
  Pipe2/1(Outflow) -> Sum1/1
  Saturation2/1 -> f_2(y,u)/1
  Ground/1 -> Pipe3/2(Level 2)
  u_2/1 -> Sum1/2
  Gain2/1 -> Sum1/3
  Pipe3/1(Outflow) -> Gain2/1
  Sum2/1 -> Saturation2/1
  Sum1/1 -> Tank 2 Section/1  "flow to tank 2"
  y_3/1 -> Pipe2/1(Level 1)

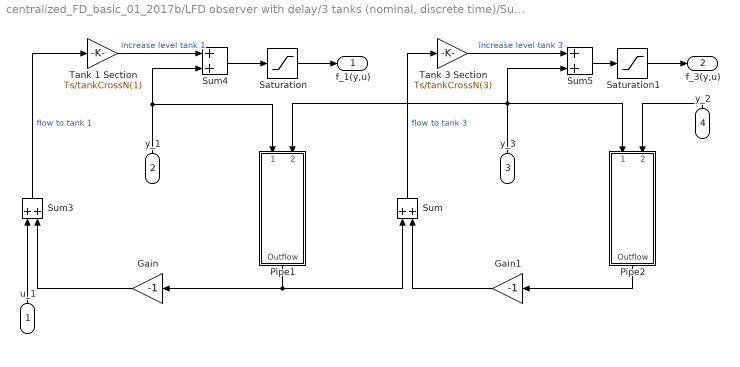
== system centralized_FD_basic_01_2017b/LFD observer with delay/3 tanks (nominal, discrete time)/Subsystem ==
  u_1 : Inport
  y_1 : Inport  Port=2
  y_3 : Inport  Port=3
  y_2 : Inport  Port=4
  Gain : Gain  Gain=-1
  Gain1 : Gain  Gain=-1
  Pipe1 : Subsystem  mask(Connection Pipe){S_p=pipeCrossN(1), c_o=pipeCoeffN(1)}
      mask prompts: S_p "Pipe cross-section [m^2]"; c_o "Outflow coefficient"
      mask help:
      | Connection pipe between two tanks.
      | The pipe cross-section and the outflow coefficient are mask block parameters.
      mask Help:
      | Enter the pipe cross-section [S_p] and the outflow coefficient [c_o] in the block dialog parameter fields.
      | 
      | The block generates the pipe's flow-rate. The input signals are the level of fluid into both the tanks, connected by the pipe. If the level in the first tank is bigger than the level in the second one, the fluid flow from the first to the second tank, else in the opposite way.
      mask Display: image(imread('pipe.jpg'));
  Pipe2 : Subsystem  mask(Connection Pipe){S_p=pipeCrossN(2), c_o=pipeCoeffN(2)}
      mask prompts: S_p "Pipe cross-section [m^2]"; c_o "Outflow coefficient"
      mask help:
      | Connection pipe between two tanks.
      | The pipe cross-section and the outflow coefficient are mask block parameters.
      mask Help:
      | Enter the pipe cross-section [S_p] and the outflow coefficient [c_o] in the block dialog parameter fields.
      | 
      | The block generates the pipe's flow-rate. The input signals are the level of fluid into both the tanks, connected by the pipe. If the level in the first tank is bigger than the level in the second one, the fluid flow from the first to the second tank, else in the opposite way.
      mask Display: image(imread('pipe.jpg'));
  Saturation : Saturate  UpperLimit=tankMaxN(1)  LowerLimit=tankMinN(1)
  Saturation1 : Saturate  UpperLimit=tankMaxN(3)  LowerLimit=tankMinN(3)
  Sum{,3..5} (4 alike) : Sum
  Tank 1 Section : Gain  Gain=Ts/tankCrossN(1)  SaturateOnIntegerOverflow=on  OutDataTypeStr=Inherit: Same as input  ParamDataTypeStr=Inherit: Same as input
  Tank 3 Section : Gain  Gain=Ts/tankCrossN(3)  SaturateOnIntegerOverflow=on  OutDataTypeStr=Inherit: Same as input  ParamDataTypeStr=Inherit: Same as input
  f_1(y,u) : Outport
  f_3(y,u) : Outport  Port=2
  wires:
  Saturation1/1 -> f_3(y,u)/1
  Sum3/1 -> Tank 1 Section/1  "flow to tank 1"
  y_2/1 -> Pipe2/2(Level 2)
  Pipe2/1(Outflow) -> Gain1/1
  Tank 3 Section/1 -> Sum5/1  "increase level tank 3"
  Pipe1/1(Outflow) -> Sum/1, Gain/1
  Tank 1 Section/1 -> Sum4/1  "increase level tank 1"
  u_1/1 -> Sum3/1
  Saturation/1 -> f_1(y,u)/1
  Gain/1 -> Sum3/2
  Sum4/1 -> Saturation/1
  y_1/1 -> Pipe1/1(Level 1), Sum4/2
  Sum5/1 -> Saturation1/1
  Sum/1 -> Tank 3 Section/1  "flow to tank 3"
  Gain1/1 -> Sum/2
  y_3/1 -> Pipe2/1(Level 1), Sum5/2, Pipe1/2(Level 2)

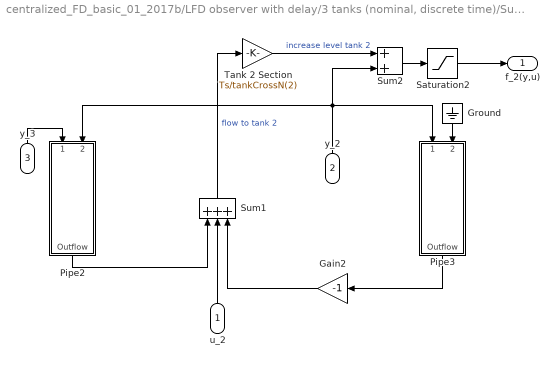
== system centralized_FD_basic_01_2017b/LFD observer with delay/3 tanks (nominal, discrete time)/Subsystem1 ==
  u_2 : Inport
  y_2 : Inport  Port=2
  y_3 : Inport  Port=3
  Gain2 : Gain  Gain=-1
  Ground : Ground
  Pipe2 : Subsystem  mask(Connection Pipe){S_p=pipeCrossN(2), c_o=pipeCoeffN(2)}
      mask prompts: S_p "Pipe cross-section [m^2]"; c_o "Outflow coefficient"
      mask help:
      | Connection pipe between two tanks.
      | The pipe cross-section and the outflow coefficient are mask block parameters.
      mask Help:
      | Enter the pipe cross-section [S_p] and the outflow coefficient [c_o] in the block dialog parameter fields.
      | 
      | The block generates the pipe's flow-rate. The input signals are the level of fluid into both the tanks, connected by the pipe. If the level in the first tank is bigger than the level in the second one, the fluid flow from the first to the second tank, else in the opposite way.
      mask Display: image(imread('pipe.jpg'));
  Pipe3 : Subsystem  mask(Connection Pipe){S_p=pipeCrossN(3), c_o=pipeCoeffN(3)}
      mask prompts: S_p "Pipe cross-section [m^2]"; c_o "Outflow coefficient"
      mask help:
      | Connection pipe between two tanks.
      | The pipe cross-section and the outflow coefficient are mask block parameters.
      mask Help:
      | Enter the pipe cross-section [S_p] and the outflow coefficient [c_o] in the block dialog parameter fields.
      | 
      | The block generates the pipe's flow-rate. The input signals are the level of fluid into both the tanks, connected by the pipe. If the level in the first tank is bigger than the level in the second one, the fluid flow from the first to the second tank, else in the opposite way.
      mask Display: image(imread('pipe.jpg'));
  Saturation2 : Saturate  UpperLimit=tankMaxN(2)  LowerLimit=tankMinN(2)
  Sum1 : Sum  Inputs=+++
  Sum2 : Sum
  Tank 2 Section : Gain  Gain=Ts/tankCrossN(2)  SaturateOnIntegerOverflow=on  OutDataTypeStr=Inherit: Same as input  ParamDataTypeStr=Inherit: Same as input
  f_2(y,u) : Outport
  wires:
  Tank 2 Section/1 -> Sum2/1  "increase level tank 2"
  y_2/1 -> Pipe2/2(Level 2), Sum2/2, Pipe3/1(Level 1)
  Pipe2/1(Outflow) -> Sum1/1
  Saturation2/1 -> f_2(y,u)/1
  Ground/1 -> Pipe3/2(Level 2)
  u_2/1 -> Sum1/2
  Gain2/1 -> Sum1/3
  Pipe3/1(Outflow) -> Gain2/1
  Sum2/1 -> Saturation2/1
  Sum1/1 -> Tank 2 Section/1  "flow to tank 2"
  y_3/1 -> Pipe2/1(Level 1)

== system centralized_FD_basic_01_2017b/LFD observer no delay/3 tanks (nominal, discrete time)/Subsystem/Pipe1 ==
  Level 1 : Inport
  Level 2 : Inport  Port=2
  2g : Gain  Gain=2*9.8  SaturateOnIntegerOverflow=on  OutDataTypeStr=Inherit: Same as input  ParamDataTypeStr=Inherit: Same as input
  Abs : Abs  SaturateOnIntegerOverflow=on
  Math Function : Math  Operator=sqrt  SaturateOnIntegerOverflow=on
  Pipe Section : Gain  Gain=S_p  SaturateOnIntegerOverflow=on  OutDataTypeStr=Inherit: Same as input  ParamDataTypeStr=Inherit: Same as input
  Product : Product  SaturateOnIntegerOverflow=on  InputSameDT=on  OutDataTypeStr=Inherit: Same as first input
  Sign : Signum
  Sum : Sum  Inputs=+-  SaturateOnIntegerOverflow=on  InputSameDT=on  OutDataTypeStr=Inherit: Same as first input
  outflow coeff. : Gain  Gain=c_o  SaturateOnIntegerOverflow=on  OutDataTypeStr=Inherit: Same as input  ParamDataTypeStr=Inherit: Same as input
  Outflow : Outport
  wires:
  outflow coeff./1 -> Outflow/1
  Pipe Section/1 -> outflow coeff./1
  Product/1 -> Pipe Section/1
  Sign/1 -> Product/1
  Math Function/1 -> Product/2
  2g/1 -> Math Function/1
  Abs/1 -> 2g/1
  Sum/1 -> Abs/1, Sign/1
  Level 2/1 -> Sum/2
  Level 1/1 -> Sum/1

== system centralized_FD_basic_01_2017b/LFD observer no delay/3 tanks (nominal, discrete time)/Subsystem/Pipe2 ==
  Level 1 : Inport
  Level 2 : Inport  Port=2
  2g : Gain  Gain=2*9.8  SaturateOnIntegerOverflow=on  OutDataTypeStr=Inherit: Same as input  ParamDataTypeStr=Inherit: Same as input
  Abs : Abs  SaturateOnIntegerOverflow=on
  Math Function : Math  Operator=sqrt  SaturateOnIntegerOverflow=on
  Pipe Section : Gain  Gain=S_p  SaturateOnIntegerOverflow=on  OutDataTypeStr=Inherit: Same as input  ParamDataTypeStr=Inherit: Same as input
  Product : Product  SaturateOnIntegerOverflow=on  InputSameDT=on  OutDataTypeStr=Inherit: Same as first input
  Sign : Signum
  Sum : Sum  Inputs=+-  SaturateOnIntegerOverflow=on  InputSameDT=on  OutDataTypeStr=Inherit: Same as first input
  outflow coeff. : Gain  Gain=c_o  SaturateOnIntegerOverflow=on  OutDataTypeStr=Inherit: Same as input  ParamDataTypeStr=Inherit: Same as input
  Outflow : Outport
  wires:
  outflow coeff./1 -> Outflow/1
  Pipe Section/1 -> outflow coeff./1
  Product/1 -> Pipe Section/1
  Sign/1 -> Product/1
  Math Function/1 -> Product/2
  2g/1 -> Math Function/1
  Abs/1 -> 2g/1
  Sum/1 -> Abs/1, Sign/1
  Level 2/1 -> Sum/2
  Level 1/1 -> Sum/1

== system centralized_FD_basic_01_2017b/LFD observer no delay/3 tanks (nominal, discrete time)/Subsystem1/Pipe2 ==
  Level 1 : Inport
  Level 2 : Inport  Port=2
  2g : Gain  Gain=2*9.8  SaturateOnIntegerOverflow=on  OutDataTypeStr=Inherit: Same as input  ParamDataTypeStr=Inherit: Same as input
  Abs : Abs  SaturateOnIntegerOverflow=on
  Math Function : Math  Operator=sqrt  SaturateOnIntegerOverflow=on
  Pipe Section : Gain  Gain=S_p  SaturateOnIntegerOverflow=on  OutDataTypeStr=Inherit: Same as input  ParamDataTypeStr=Inherit: Same as input
  Product : Product  SaturateOnIntegerOverflow=on  InputSameDT=on  OutDataTypeStr=Inherit: Same as first input
  Sign : Signum
  Sum : Sum  Inputs=+-  SaturateOnIntegerOverflow=on  InputSameDT=on  OutDataTypeStr=Inherit: Same as first input
  outflow coeff. : Gain  Gain=c_o  SaturateOnIntegerOverflow=on  OutDataTypeStr=Inherit: Same as input  ParamDataTypeStr=Inherit: Same as input
  Outflow : Outport
  wires:
  outflow coeff./1 -> Outflow/1
  Pipe Section/1 -> outflow coeff./1
  Product/1 -> Pipe Section/1
  Sign/1 -> Product/1
  Math Function/1 -> Product/2
  2g/1 -> Math Function/1
  Abs/1 -> 2g/1
  Sum/1 -> Abs/1, Sign/1
  Level 2/1 -> Sum/2
  Level 1/1 -> Sum/1

== system centralized_FD_basic_01_2017b/LFD observer no delay/3 tanks (nominal, discrete time)/Subsystem1/Pipe3 ==
  Level 1 : Inport
  Level 2 : Inport  Port=2
  2g : Gain  Gain=2*9.8  SaturateOnIntegerOverflow=on  OutDataTypeStr=Inherit: Same as input  ParamDataTypeStr=Inherit: Same as input
  Abs : Abs  SaturateOnIntegerOverflow=on
  Math Function : Math  Operator=sqrt  SaturateOnIntegerOverflow=on
  Pipe Section : Gain  Gain=S_p  SaturateOnIntegerOverflow=on  OutDataTypeStr=Inherit: Same as input  ParamDataTypeStr=Inherit: Same as input
  Product : Product  SaturateOnIntegerOverflow=on  InputSameDT=on  OutDataTypeStr=Inherit: Same as first input
  Sign : Signum
  Sum : Sum  Inputs=+-  SaturateOnIntegerOverflow=on  InputSameDT=on  OutDataTypeStr=Inherit: Same as first input
  outflow coeff. : Gain  Gain=c_o  SaturateOnIntegerOverflow=on  OutDataTypeStr=Inherit: Same as input  ParamDataTypeStr=Inherit: Same as input
  Outflow : Outport
  wires:
  outflow coeff./1 -> Outflow/1
  Pipe Section/1 -> outflow coeff./1
  Product/1 -> Pipe Section/1
  Sign/1 -> Product/1
  Math Function/1 -> Product/2
  2g/1 -> Math Function/1
  Abs/1 -> 2g/1
  Sum/1 -> Abs/1, Sign/1
  Level 2/1 -> Sum/2
  Level 1/1 -> Sum/1

== system centralized_FD_basic_01_2017b/LFD observer with delay/3 tanks (nominal, discrete time)/Subsystem/Pipe1 ==
  Level 1 : Inport
  Level 2 : Inport  Port=2
  2g : Gain  Gain=2*9.8  SaturateOnIntegerOverflow=on  OutDataTypeStr=Inherit: Same as input  ParamDataTypeStr=Inherit: Same as input
  Abs : Abs  SaturateOnIntegerOverflow=on
  Math Function : Math  Operator=sqrt  SaturateOnIntegerOverflow=on
  Pipe Section : Gain  Gain=S_p  SaturateOnIntegerOverflow=on  OutDataTypeStr=Inherit: Same as input  ParamDataTypeStr=Inherit: Same as input
  Product : Product  SaturateOnIntegerOverflow=on  InputSameDT=on  OutDataTypeStr=Inherit: Same as first input
  Sign : Signum
  Sum : Sum  Inputs=+-  SaturateOnIntegerOverflow=on  InputSameDT=on  OutDataTypeStr=Inherit: Same as first input
  outflow coeff. : Gain  Gain=c_o  SaturateOnIntegerOverflow=on  OutDataTypeStr=Inherit: Same as input  ParamDataTypeStr=Inherit: Same as input
  Outflow : Outport
  wires:
  outflow coeff./1 -> Outflow/1
  Pipe Section/1 -> outflow coeff./1
  Product/1 -> Pipe Section/1
  Sign/1 -> Product/1
  Math Function/1 -> Product/2
  2g/1 -> Math Function/1
  Abs/1 -> 2g/1
  Sum/1 -> Abs/1, Sign/1
  Level 2/1 -> Sum/2
  Level 1/1 -> Sum/1
